simulink model "ex8_2"  (R2015a)
settings: Solver=ode45  SolverMode=SingleTasking  StartTime=0.0  StopTime=.6  RelTol=1e-5
libraries: powerlib x17, powerlib_meascontrol x4
settings Model: CovMetricSettings=dwe  CovHtmlReporting=off  covSaveCumulativeToWorkspaceVar=off  CovSaveSingleToWorkspaceVar=off  CovExternalEMLEnable=on  Creator=Omid  LastModifiedBy=Omid
settings SolverCC: ZeroCrossAlgorithm=Adaptive
settings DataIOCC: LimitDataPoints=off  SaveFormat=Dataset  ReturnWorkspaceOutputs=on
settings DebuggingCC: IgnoredZcDiagnostic=none  UnconnectedInputMsg=none  UnconnectedOutputMsg=none  UnconnectedLineMsg=none  SFUnexpectedBacktrackingDiag=error  SFNoUnconditionalDefaultTransitionDiag=error
settings HardwareCC: ProdBitPerPointer=64  ProdLargestAtomicFloat=Float  ProdIntDivRoundTo=Zero  ProdEndianess=LittleEndian  ProdHWDeviceType=Specified
settings ModelReferenceCC: PropagateSignalLabelsOutOfModel=on
settings SFSimCC: SimUseLocalCustomCode=on
settings RTWCC: RTWUseLocalCustomCode=on
settings GRTTargetCC: TargetLangStandard=C99 (ISO)
settings ConfigurationSet: Description=Simscape Multibody

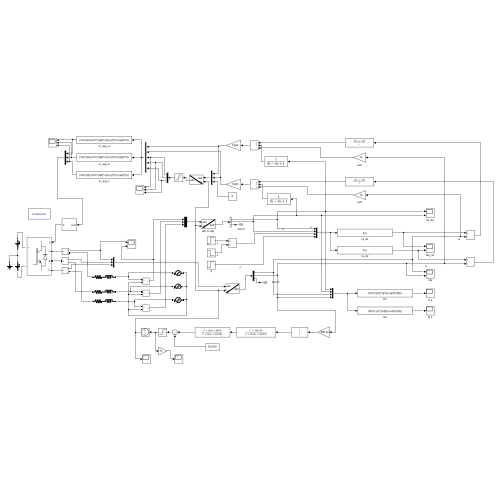
[thumbnail: Simulink's stored preview of the top-level diagram]
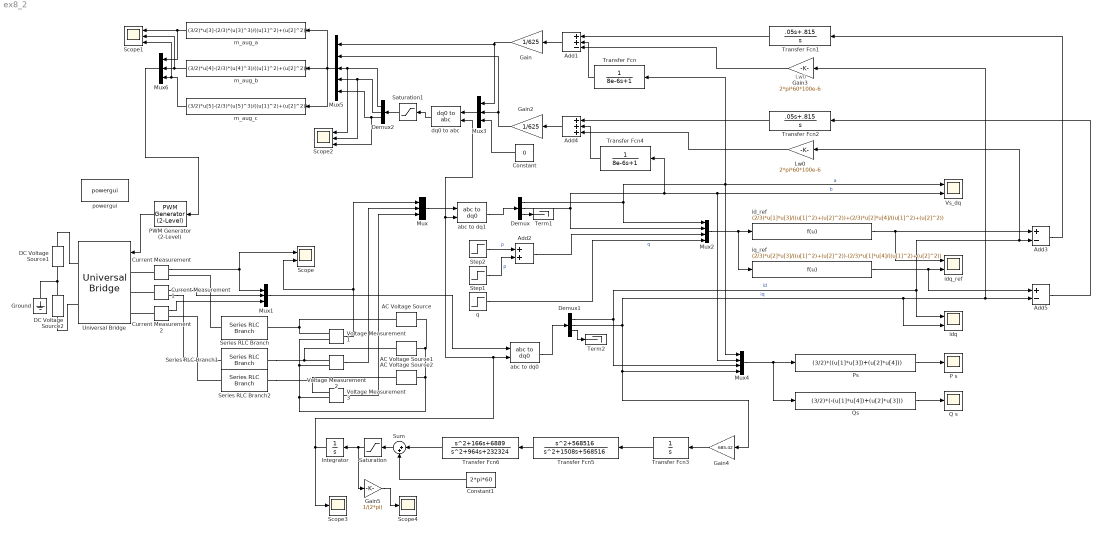
== system ex8_2 ==
  note: Lw0
  AC Voltage Source : powerlib/Electrical Sources/AC Voltage Source  Amplitude=391  Phase=90  Frequency=60  SampleTime=0  Measurements=None  BusType=swing  Pref=10e3  Qref=0  Qmin=-inf  Qmax=+inf
  AC Voltage Source1 : powerlib/Electrical Sources/AC Voltage Source  Amplitude=391  Phase=-30  Frequency=60  SampleTime=0  Measurements=None  BusType=swing  Pref=10e3  Qref=0  Qmin=-inf  Qmax=+inf
  AC Voltage Source2 : powerlib/Electrical Sources/AC Voltage Source  Amplitude=391  Phase=-150  Frequency=60  SampleTime=0  Measurements=None  BusType=swing  Pref=10e3  Qref=0  Qmin=-inf  Qmax=+inf
  Add1 : Sum  Inputs=++-
  Add2 : Sum
  Add3 : Sum  Inputs=+-
  Add4 : Sum  Inputs=+++
  Add5 : Sum  Inputs=+-
  Constant : Constant  Value=0
  Constant1 : Constant  Value=2*pi*60
  Current Measurement : powerlib/Measurements/Current Measurement  PhasorSimulation=off  OutputType=Complex  PSBequivalent=0
  Current Measurement1 : powerlib/Measurements/Current Measurement  PhasorSimulation=off  OutputType=Complex  PSBequivalent=0
  Current Measurement2 : powerlib/Measurements/Current Measurement  PhasorSimulation=off  OutputType=Complex  PSBequivalent=0
  DC Voltage Source1 : powerlib/Electrical Sources/DC Voltage Source  Amplitude=625  Measurements=None
  DC Voltage Source2 : powerlib/Electrical Sources/DC Voltage Source  Amplitude=625  Measurements=None
  Demux : Demux  Outputs=3
      settings: DisplayOption=none
  Demux1 : Demux  Outputs=3
  Demux2 : Demux  Outputs=3
  Gain : Gain  Gain=1/625
  Gain2 : Gain  Gain=1/625
  Gain3 : Gain  Gain=2*pi*60*100e-6
  Gain4 : Gain  Gain=685.42
  Gain5 : Gain  Gain=1/(2*pi)
  Ground : powerlib/Elements/Ground  LConnTagsString=a
  Integrator : Integrator  WrapState=on  WrappedStateUpperValue=pi*2  WrappedStateLowerValue=0
  Lw0 : Gain  Gain=2*pi*60*100e-6
  Mux{,1,3,6} (4 alike) : Mux  Inputs=3
  Mux2 : Mux
  Mux4 : Mux
  Mux5 : Mux  Inputs=5
  P s : Scope
      settings: TimeRange=auto  MaxDataPoints=5000  SaveToWorkspace=off  SaveName=ScopeData4  YMin=-3252134.85809  YMax=3281324.09692  SampleTime=-1
  PWM Generator (2-Level) : powerlib_meascontrol/Pulse & Signal Generators/PWM Generator (2-Level)  ModulatorType=Three-phase bridge (6 pulses)  ModulatorMode=Unsynchronized  Fc=3420  Pc=90  nF=27  MinMax="[ -1  1 ]"  SamplingTechnique=Natural  ModulatingSignals=off  m=0.8  Freq=60  Phase=0  Ts=0  ShowCarrierOutport=off
  Ps : Fcn  Expr=(3/2)*((u[1]*u[3])+(u[2]*u[4]))
  Q s : Scope
      settings: TimeRange=auto  MaxDataPoints=5000  SaveToWorkspace=off  SaveName=ScopeData5  YMin=-326223.55067  YMax=1295625.37251  SampleTime=-1
  Qs : Fcn  Expr=(3/2)*(-(u[1]*u[4])+(u[2]*u[3]))
  Saturation : Saturate  UpperLimit=2*pi*75  LowerLimit=2*pi*55
  Saturation1 : Saturate  UpperLimit=1  LowerLimit=-1
  Scope : Scope  NumInputPorts=2
      settings: TimeRange=auto  MaxDataPoints=5000  SaveToWorkspace=off  SaveName=ScopeData  YMin=-5830.82428~-5  YMax=5833.60919~5  SampleTime=-1
  Scope1 : Scope  NumInputPorts=3
      settings: TimeRange=auto  MaxDataPoints=5000  SaveToWorkspace=off  YMin=-1.07225~-5~-5  YMax=1.07228~5~5  SampleTime=-1
  Scope2 : Scope  NumInputPorts=3
      settings: TimeRange=auto  MaxDataPoints=5000  SaveToWorkspace=off  SaveName=ScopeData2  YMin=-0.79956~-5~-5  YMax=0.79799~5~5  SampleTime=-1
  Scope3 : Scope
      settings: TimeRange=auto  MaxDataPoints=5000  SaveToWorkspace=off  YMin=-0.78454  YMax=7.0609  SampleTime=-1
  Scope4 : Scope
      settings: TimeRange=auto  MaxDataPoints=5000  SaveToWorkspace=off  SaveName=ScopeData2  YMin=52.5  YMax=77.5  SampleTime=-1
  Series RLC Branch : powerlib/Elements/Series RLC Branch  LConnTagsString=__new0  RConnTagsString=__new0  BranchType=RL  Resistance=.00075  Inductance=100e-6  SetiL0=off  InitialCurrent=1600  Capacitance=1e-6  Setx0=off  InitialVoltage=0  Measurements=None
  Series RLC Branch1 : powerlib/Elements/Series RLC Branch  LConnTagsString=__new0  RConnTagsString=__new0  BranchType=RL  Resistance=.00075  Inductance=100e-6  SetiL0=off  InitialCurrent=1600  Capacitance=1e-6  Setx0=off  InitialVoltage=0  Measurements=None
  Series RLC Branch2 : powerlib/Elements/Series RLC Branch  LConnTagsString=__new0  RConnTagsString=__new0  BranchType=RL  Resistance=.00075  Inductance=100e-6  SetiL0=off  InitialCurrent=1600  Capacitance=1e-6  Setx0=off  InitialVoltage=0  Measurements=None
  Step1 : Step  Time=.3  After=-5e6  SampleTime=0
  Step2 : Step  Time=.2  After=2.5e6  SampleTime=0
  Sum : Sum  Inputs=|++
  Term1 : Terminator
  Term2 : Terminator
  Transfer Fcn : TransferFcn  Denominator=[8e-6 1]
  Transfer Fcn1 : TransferFcn  Numerator=[.05 .815]  Denominator=[1 0]
  Transfer Fcn2 : TransferFcn  Numerator=[.05 .815]  Denominator=[1 0]
  Transfer Fcn3 : TransferFcn  Denominator=[1 0]
  Transfer Fcn4 : TransferFcn  Denominator=[8e-6 1]
  Transfer Fcn5 : TransferFcn  Numerator=[1 0 568516]  Denominator=[1 1508 568516]
  Transfer Fcn6 : TransferFcn  Numerator=[1 166 6889]  Denominator=[1 964 232324]
  Universal Bridge : powerlib/Power Electronics/Universal Bridge  Arms=3  SnubberResistance=1e5  SnubberCapacitance=inf  Device=IGBT / Diodes  Ron=.88e-3  Lon=0  ForwardVoltages="[  1  1 ]"  ForwardVoltage=0  GTOparameters=[ 10e-6 , 20e-6 ]  IGBTparameters=[ 1e-6 , 2e-6 ]  Measurements=None  Measurements_2=None  converterType=Rectifier
  Voltage Measurement1 : powerlib/Measurements/Voltage Measurement  PhasorSimulation=off  OutputType=Complex  PSBequivalent=0
  Voltage Measurement2 : powerlib/Measurements/Voltage Measurement  PhasorSimulation=off  OutputType=Complex  PSBequivalent=0
  Voltage Measurement3 : powerlib/Measurements/Voltage Measurement  PhasorSimulation=off  OutputType=Complex  PSBequivalent=0
  "Vs_dq " : Scope  NumInputPorts=2
      settings: TimeRange=auto  MaxDataPoints=5000  SaveToWorkspace=off  SaveName=ScopeData3  YMin=-2483.2971~-5  YMax=2875.43543~5  SampleTime=-1
  abc to dq0 : powerlib_meascontrol/Transformations/abc to dq0  Alignment=90 degrees behind phase A axis
  abc to dq1 : powerlib_meascontrol/Transformations/abc to dq0  Alignment=90 degrees behind phase A axis
  dq0 to abc : powerlib_meascontrol/Transformations/dq0 to abc  Alignment=90 degrees behind phase A axis
  id_ref : Fcn  Expr=(2/3)*u[1]*u[3]/((u[1]^2)+(u[2]^2))+(2/3)*u[2]*u[4]/((u[1]^2)+(u[2]^2))
  idq : Scope  NumInputPorts=2
      settings: TimeRange=auto  MaxDataPoints=5000  SaveToWorkspace=off  SaveName=ScopeData2  YMin=-5471.00825~-5  YMax=5915.00839~5  SampleTime=-1
  idq_ref : Scope  NumInputPorts=2
      settings: TimeRange=auto  MaxDataPoints=5000  SaveToWorkspace=off  YMin=-6000~-5  YMax=6000~5  SampleTime=-1
  iq_ref : Fcn  Expr=(2/3)*u[2]*u[3]/((u[1]^2)+(u[2]^2))-(2/3)*u[1]*u[4]/((u[1]^2)+(u[2]^2))
  m_aug_a : Fcn  Expr=(3/2)*u[3]-(2/3)*(u[3]^3)/((u[1]^2)+(u[2]^2))
  m_aug_b : Fcn  Expr=(3/2)*u[4]-(2/3)*(u[4]^3)/((u[1]^2)+(u[2]^2))
  m_aug_c : Fcn  Expr=(3/2)*u[5]-(2/3)*(u[5]^3)/((u[1]^2)+(u[2]^2))
  powergui : powerlib/powergui  Priority=1  SimulationMode=Continuous  SampleTime=50e-6  frequency=60  Iterations=50  frequencyindice=0  Pbase=100e6  ErrMax=1e-4  UnitsV=kV  UnitsW=MW  buscounter=0  FunctionMessages=off  echomessages=off  EnableUseOfTLC=off  CurrentSourceSwitches=off  DisableSnubberDevices=off  DisableRonSwitches=off  DisableVfSwitches=off  DisplayEquations=off  AutomaticDiscreteSolvers=off  SolverType=Tustin/Backward Euler (TBE)  Interpol=off  ExternalGateDelay=off  methode=off  Ts=100  x0status=blocks  SPID=on  SwTol=0  HookPort=off  NonlinearTolerance=1e-4  nMaxIteration=100  ContinueOnMaxIteration=off  RestoreLinks=warning  ResistiveCurrentMeasurement=off  Frange=[0:2:500]  Ylog=off  Xlog=on  ShowGrid=off  save=off  variable=ZData  structure=0  ZoomFFT=off  StartTime=0.0  cycles=1  DisplayStyle=1  fundamental=60  FreqAxis=off  MaxFrequency=1000  frequencyindicesteady=1  RmsSteady=1  display=off
  q : Step  Time=.35  After=1e6  SampleTime=0
  wires:
  Add1/1 -> Gain/1
  Voltage Measurement1/1 -> Mux/1, Scope/2
  Transfer Fcn/1 -> Add1/2
  Transfer Fcn1/1 -> Add1/1
  Add3/1 -> Transfer Fcn1/1
  Voltage Measurement3/1 -> Mux/3
  Voltage Measurement2/1 -> Mux/2
  Mux/1 -> abc to dq1/1
  abc to dq1/1 -> Demux/1
  abc to dq0/1 -> Demux1/1
  Mux1/1 -> abc to dq0/1
  Current Measurement1/1 -> Mux1/2
  Current Measurement2/1 -> Mux1/3
  Demux/1 -> Transfer Fcn/1, Mux4/1, "Vs_dq "/1, Mux2/1  "a"
  Demux/2 -> Transfer Fcn4/1, Mux4/2, "Vs_dq "/2, Mux2/2  "b"
  q/1 -> Mux2/4  "q"
  Mux2/1 -> id_ref/1, iq_ref/1
  id_ref/1 -> Add3/1, idq_ref/1
  Demux1/1 -> idq/1, Add3/2, Lw0/1, Mux4/3  "id"
  Transfer Fcn2/1 -> Add4/1
  Transfer Fcn4/1 -> Add4/2
  Add4/1 -> Gain2/1
  Add5/1 -> Transfer Fcn2/1
  iq_ref/1 -> idq_ref/2, Add5/1
  Demux1/2 -> Gain4/1, Mux4/4, idq/2, Gain3/1, Add5/2  "iq"
  dq0 to abc/1 -> Saturation1/1
  Gain2/1 -> Mux3/2, Mux5/2
  Gain/1 -> Mux3/1, Mux5/1
  PWM Generator (2-Level)/1 -> Universal Bridge/1
  Mux3/1 -> dq0 to abc/1
  Constant/1 -> Mux3/3
  Current Measurement/1 -> Mux1/1, Scope/1
  Demux1/3 -> Term2/1
  Demux/3 -> Term1/1
  Mux4/1 -> Qs/1, Ps/1
  Ps/1 -> P s/1
  Qs/1 -> Q s/1
  Demux2/1 -> Mux5/3, Scope2/1
  Demux2/2 -> Scope2/2, Mux5/4
  Demux2/3 -> Scope2/3, Mux5/5
  Mux5/1 -> m_aug_a/1, m_aug_b/1, m_aug_c/1
  m_aug_c/1 -> Scope1/3, Mux6/3
  Saturation1/1 -> Demux2/1
  Mux6/1 -> PWM Generator (2-Level)/1
  m_aug_a/1 -> Mux6/1, Scope1/1
  m_aug_b/1 -> Scope1/2, Mux6/2
  Step2/1 -> Add2/1  "p"
  Step1/1 -> Add2/2  "p"
  Add2/1 -> Mux2/3
  Gain3/1 -> Add1/3
  Lw0/1 -> Add4/3
  Transfer Fcn3/1 -> Transfer Fcn5/1
  Gain4/1 -> Transfer Fcn3/1
  Gain5/1 -> Scope4/1
  Saturation/1 -> Gain5/1, Integrator/1
  Transfer Fcn5/1 -> Transfer Fcn6/1
  Sum/1 -> Saturation/1
  Integrator/1 -> Scope3/1, abc to dq1/2, dq0 to abc/2, abc to dq0/2
  Constant1/1 -> Sum/2
  Transfer Fcn6/1 -> Sum/1
  connections:
  DC Voltage Source1/RConn1 -- Universal Bridge/RConn1
  Current Measurement/LConn1 -- Universal Bridge/LConn1
  Series RLC Branch/LConn1 -- Current Measurement/RConn1
  Voltage Measurement1/LConn1 -- AC Voltage Source/RConn1 -- Series RLC Branch/RConn1
  Current Measurement1/LConn1 -- Universal Bridge/LConn2
  Current Measurement1/RConn1 -- Series RLC Branch1/LConn1
  Voltage Measurement2/LConn1 -- Series RLC Branch1/RConn1 -- AC Voltage Source1/RConn1
  Current Measurement2/LConn1 -- Universal Bridge/LConn3
  Series RLC Branch2/LConn1 -- Current Measurement2/RConn1
  AC Voltage Source2/RConn1 -- Series RLC Branch2/RConn1 -- Voltage Measurement3/LConn1
  DC Voltage Source2/LConn1 -- Universal Bridge/RConn2
  DC Voltage Source2/RConn1 -- Ground/LConn1 -- DC Voltage Source1/LConn1
  Voltage Measurement2/LConn2 -- AC Voltage Source/LConn1 -- AC Voltage Source1/LConn1 -- AC Voltage Source2/LConn1 -- Voltage Measurement3/LConn2 -- Voltage Measurement1/LConn2
